simulink model "JointSpaceInverseDynamic"  (R2020a)
settings: Solver=VariableStepAuto  StartTime=0.0  StopTime=2.0  RelTol=1e-3
values from neighbouring files (symbols this model uses):
  g = 9.81    [params.m]
  KD = diag([ 24  24  24])    [params.m]
  KP = diag([200 200 200])    [params.m]
  traj_on = 1    [params.m]
libraries: robotcorelib x1, simulink x1, vrlib x1
settings Model: Creator=Sebastiano  LastModifiedBy=Sebastiano

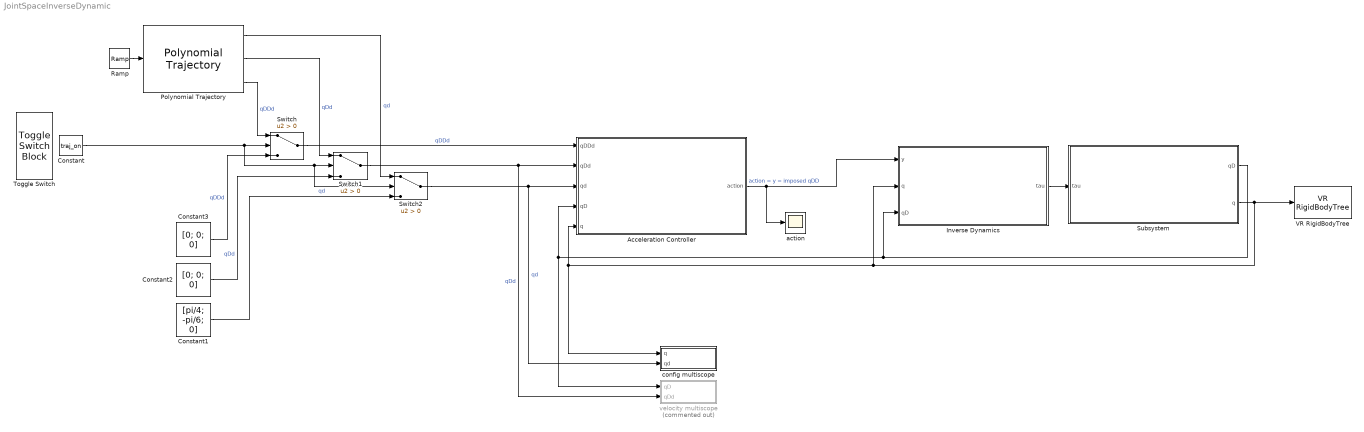
== system JointSpaceInverseDynamic ==
  Acceleration Controller : Subsystem
  Constant : Constant  Value=traj_on
  Constant1 : Constant  Value=[pi/4; -pi/6; 0]  VectorParams1D=off
  Constant2 : Constant  Value=[0; 0; 0]  VectorParams1D=off
  Constant3 : Constant  Value=[0; 0; 0]  VectorParams1D=off
  Inverse Dynamics : Subsystem
  Polynomial Trajectory : robotcorelib/Polynomial Trajectory  WaypointSource=Internal  Waypoints=[ pi/4, -pi/2, pi/4; -pi/4, pi/4, -pi/6; 0.1, -0.1, 0.2]  TimePoints=[ 0, 1.5, 2 ]  TimeInterval=[ 1, 4 ]  Method=Cubic Polynomial  ParameterSource=Internal  VelocityBoundaryCondition=zeros( 3, 3 )  AccelerationBoundaryCondition=zeros( 2, 5 )  SimulateUsing=Interpreted execution
      settings: SourceProductBaseCode=NV,RO,RR
  Ramp : simulink/Sources/Ramp  slope=1  start=0  InitialOutput=0
  Subsystem : Subsystem
  Switch : Switch  Criteria=u2 > Threshold
  Switch1 : Switch  Criteria=u2 > Threshold
  Switch2 : Switch  Criteria=u2 > Threshold
  Toggle Switch : ToggleSwitchBlock  LabelPosition=Hide
      settings: Values={{'Steady-State', 'Trajectory'}, [0 1]}
  VR RigidBodyTree : vrlib/VR RigidBodyTree  RBT=robot  useRBT=on  Ts=-1  ForceViewerOpen=on
      settings: SourceProductBaseCode=SL
  action : Scope
  config multiscope : Subsystem
  velocity multiscope : Subsystem  Commented=on
  wires:
  Acceleration Controller/1(action) -> Inverse Dynamics/1(y), action/1  "action = y = imposed qDD"
  Switch/1 -> Acceleration Controller/1(qDDd)  "qDDd"
  Switch1/1 -> velocity multiscope/2(qDd), Acceleration Controller/2(qDd)  "qDd"
  Switch2/1 -> config multiscope/2(qd), Acceleration Controller/3(qd)  "qd"
  Subsystem/2(q) -> config multiscope/1(q), Acceleration Controller/5(q), Inverse Dynamics/2(q), VR RigidBodyTree/1
  Subsystem/1(qD) -> Inverse Dynamics/3(qD), velocity multiscope/1(qD), Acceleration Controller/4(qD)
  Inverse Dynamics/1(tau) -> Subsystem/1(tau)
  Ramp/1 -> Polynomial Trajectory/1
  Polynomial Trajectory/1 -> Switch2/1  "qd"
  Polynomial Trajectory/2 -> Switch1/1  "qDd"
  Polynomial Trajectory/3 -> Switch/1  "qDDd"
  Constant3/1 -> Switch/3  "qDDd"
  Constant2/1 -> Switch1/3  "qDd"
  Constant1/1 -> Switch2/3  "qd"
  Constant/1 -> Switch2/2, Switch1/2, Switch/2

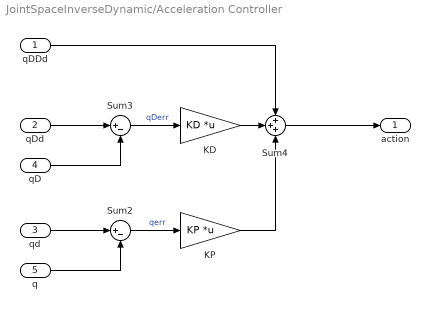
== system JointSpaceInverseDynamic/Acceleration Controller ==
  qDDd : Inport
  qDd : Inport  Port=2
  qd : Inport  Port=3
  qD : Inport  Port=4
  q : Inport  Port=5
  KD : Gain  Gain=KD  Multiplication=Matrix(K*u) (u vector)
  KP : Gain  Gain=KP  Multiplication=Matrix(K*u) (u vector)
  Sum2 : Sum  Inputs=|+-
  Sum3 : Sum  Inputs=|+-
  Sum4 : Sum  Inputs=+++
  action : Outport
  wires:
  qDd/1 -> Sum3/1
  KD/1 -> Sum4/2
  KP/1 -> Sum4/3
  qD/1 -> Sum3/2
  Sum3/1 -> KD/1  "qDerr"
  Sum4/1 -> action/1
  Sum2/1 -> KP/1  "qerr"
  qd/1 -> Sum2/1
  qDDd/1 -> Sum4/1
  q/1 -> Sum2/2

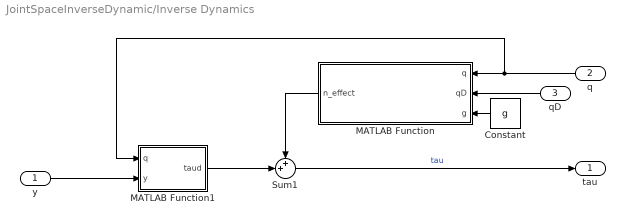
== system JointSpaceInverseDynamic/Inverse Dynamics ==
  y : Inport
  q : Inport  Port=2
  qD : Inport  Port=3
  Constant : Constant  Value=g
  MATLAB Function : MATLAB Function  TreatAsAtomicUnit=on
  MATLAB Function1 : MATLAB Function  TreatAsAtomicUnit=on
  Sum1 : Sum  Inputs=++|
  tau : Outport
  wires:
  qD/1 -> MATLAB Function/2(qD)
  MATLAB Function/1(n_effect) -> Sum1/1
  MATLAB Function1/1(taud) -> Sum1/2
  q/1 -> MATLAB Function/1(q), MATLAB Function1/1(q)
  Constant/1 -> MATLAB Function/3(g)
  y/1 -> MATLAB Function1/2(y)
  Sum1/1 -> tau/1  "tau"

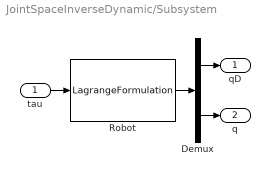
== system JointSpaceInverseDynamic/Subsystem ==
  tau : Inport
  Demux : Demux  Outputs=[3, 3]
  Robot : S-Function  FunctionName=LagrangeFormulation  Parameters=g  SFunctionDeploymentMode=off  EnableBusSupport=off
  qD : Outport
  q : Outport  Port=2
  wires:
  Robot/1 -> Demux/1
  Demux/1 -> qD/1
  tau/1 -> Robot/1
  Demux/2 -> q/1

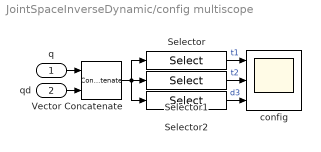
== system JointSpaceInverseDynamic/config multiscope ==
  q : Inport
  qd : Inport  Port=2
  Selector : Selector  NumberOfDimensions=2  InputPortWidth=3  IndexOptions=Index vector (dialog),Select all  Indices=1,7  OutputSizes=6,6
  Selector1 : Selector  NumberOfDimensions=2  InputPortWidth=3  IndexOptions=Index vector (dialog),Select all  Indices=2,7  OutputSizes=6,6
  Selector2 : Selector  NumberOfDimensions=2  InputPortWidth=3  IndexOptions=Index vector (dialog),Select all  Indices=3,7  OutputSizes=6,6
  Vector Concatenate : Concatenate  Mode=Multidimensional array  ConcatenateDimension=2
  config : Scope  NumInputPorts=3
  wires:
  q/1 -> Vector Concatenate/1
  qd/1 -> Vector Concatenate/2
  Selector1/1 -> config/2  "t2"
  Selector/1 -> config/1  "t1"
  Vector Concatenate/1 -> Selector/1, Selector2/1, Selector1/1
  Selector2/1 -> config/3  "d3"

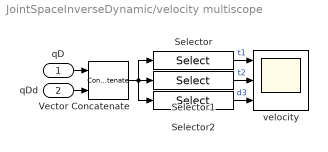
== system JointSpaceInverseDynamic/velocity multiscope ==
  qD : Inport
  qDd : Inport  Port=2
  Selector : Selector  NumberOfDimensions=2  InputPortWidth=3  IndexOptions=Index vector (dialog),Select all  Indices=1,7  OutputSizes=6,6
  Selector1 : Selector  NumberOfDimensions=2  InputPortWidth=3  IndexOptions=Index vector (dialog),Select all  Indices=2,7  OutputSizes=6,6
  Selector2 : Selector  NumberOfDimensions=2  InputPortWidth=3  IndexOptions=Index vector (dialog),Select all  Indices=3,7  OutputSizes=6,6
  Vector Concatenate : Concatenate  Mode=Multidimensional array  ConcatenateDimension=2
  velocity : Scope  NumInputPorts=3
  wires:
  qD/1 -> Vector Concatenate/1
  qDd/1 -> Vector Concatenate/2
  Selector1/1 -> velocity/2  "t2"
  Selector/1 -> velocity/1  "t1"
  Vector Concatenate/1 -> Selector/1, Selector2/1, Selector1/1
  Selector2/1 -> velocity/3  "d3"

== matlab function JointSpaceInverseDynamic/Inverse Dynamics/MATLAB Function ==
  data: q input; qD input; n_effect output; g input
function n_effect = n(q, qD, g)

n_effect = C_Lagrangian(q, qD) * qD + G_Lagrangian(q, g);

== matlab function JointSpaceInverseDynamic/Inverse Dynamics/MATLAB Function1 ==
  data: q input; taud output; y input
function taud = B(q, y)

taud = B_Lagrangian(q)*y;
